simulink model "pidsss"  (R2016a)
settings: Solver=VariableStepAuto  StartTime=0.0  StopTime=10  RelTol=1e-3
settings Model: Creator=张理官  LastModifiedBy=张理官

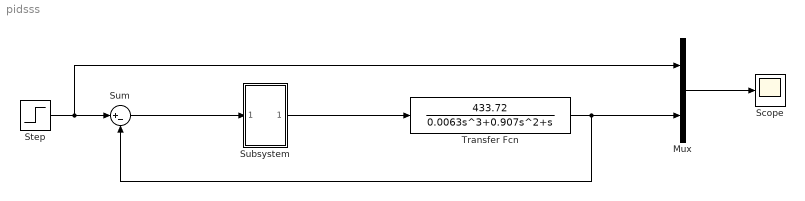
== system pidsss ==
  Mux : Mux  Inputs=2
  Scope : Scope
  Step : Step  SampleTime=0
  Subsystem : Subsystem  mask{Kp=0.33, Ki=0.3, Kd=0.063284}
      mask Display: disp('PID')
  Sum : Sum  Inputs=|+-
  Transfer Fcn : TransferFcn  Numerator=[433.72]  Denominator=[0.0063 0.907 1 0]
  wires:
  Transfer Fcn/1 -> Sum/2, Mux/2
  Mux/1 -> Scope/1
  Step/1 -> Mux/1, Sum/1
  Sum/1 -> Subsystem/1(In1)
  Subsystem/1(Out1) -> Transfer Fcn/1

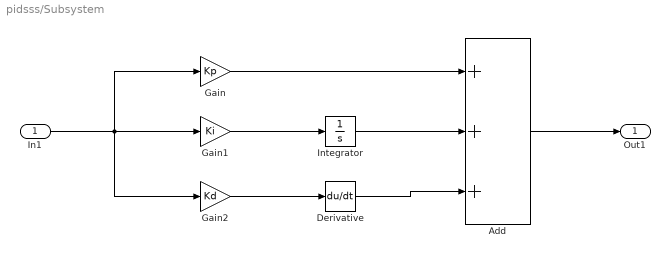
== system pidsss/Subsystem ==
  In1 : Inport
  Add : Sum  Inputs=+++
  Derivative : Derivative
  Gain : Gain  Gain=Kp
  Gain1 : Gain  Gain=Ki
  Gain2 : Gain  Gain=Kd
  Integrator : Integrator
  Out1 : Outport
  wires:
  Integrator/1 -> Add/2
  Gain/1 -> Add/1
  Derivative/1 -> Add/3
  Add/1 -> Out1/1
  Gain1/1 -> Integrator/1
  Gain2/1 -> Derivative/1
  In1/1 -> Gain2/1, Gain/1, Gain1/1
